simulink model "LMOpenLoop2"  (R2014a)
settings: Solver=ode45  StartTime=0.0  StopTime=5  MaxStep=0.0034  RelTol=1e-9
libraries: powerlib_meascontrol x2
settings Model: Creator=Daniel  LastModifiedBy=Daniel
settings SolverCC: ConsecutiveZCsStepRelTol=10*64*eps
settings DataIOCC: MaxDataPoints=200000  Refine=20

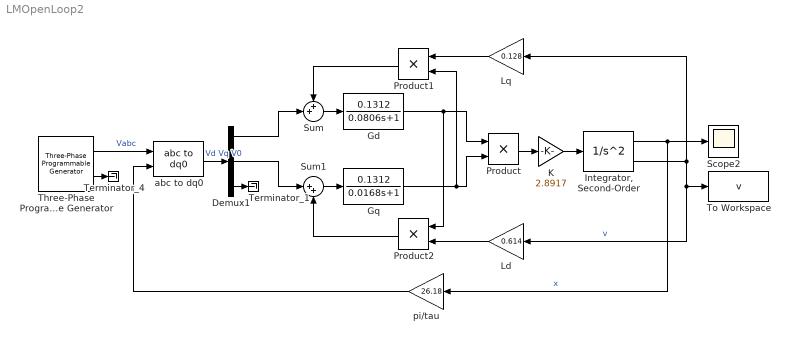
== system LMOpenLoop2 ==
  Demux1 : Demux  Outputs=3
  Gd : TransferFcn  Numerator=[0.1312]  Denominator=[0.0806 1]
  Gq : TransferFcn  Numerator=[0.1312]  Denominator=[0.0168 1]
  "Integrator, Second-Order" : SecondOrderIntegrator  ICDXDT=7.3495
  K : Gain  Gain=2.8917
  Ld : Gain  Gain=0.614
  Lq : Gain  Gain=0.128
  Product : Product
  Product1 : Product
  Product2 : Product
  Scope2 : Scope
      settings: ShowLegends=on
  Sum : Sum  Inputs=++|
  Sum1 : Sum  Inputs=|++
  Terminator_1 : Terminator
  Terminator_4 : Terminator
  Three-Phase Programmable Generator : powerlib_meascontrol/Pulse & Signal Generators/Three-Phase Programmable Generator  Par_Vps="[10.0  15  180/(2*pi)]"  VariationEntity=Amplitude  VariationType=Step  VariationStep=0  VariationRate=10  VariationMag=0.3  VariationFreq=2  Par_Timing_Variation=[0.5 1]  SinglePhase=on  Yampli=[1 0.2 1.2 1.0]  Xtime=[0 0.1 0.15 0.2]  HarmonicGeneration=off  Par_HarmoA=[1 0.3 -30 2]  Par_HarmoB=[1 0.0 0.0 1]  Par_Timing_Harmo="[0.1  1]"  Ts=50e-6
  To Workspace : ToWorkspace  VariableName=v  SaveFormat=Timeseries  SampleTime=-1
  abc to dq0 : powerlib_meascontrol/Transformations/abc to dq0  Alignment=Aligned with phase A axis
  pi/tau : Gain  Gain=26.18
  wires:
  Gd/1 -> Product/1, Product2/1
  Gq/1 -> Product1/2, Product/2
  Product/1 -> K/1
  "Integrator, Second-Order"/1 -> Scope2/1, pi/tau/1  "x"
  pi/tau/1 -> abc to dq0/2
  "Integrator, Second-Order"/2 -> To Workspace/1, Ld/1, Lq/1  "v"
  Demux1/1 -> Sum/2
  Lq/1 -> Product1/1
  Product1/1 -> Sum/1
  Sum/1 -> Gd/1
  Ld/1 -> Product2/2
  Demux1/2 -> Sum1/1
  Product2/1 -> Sum1/2
  Sum1/1 -> Gq/1
  K/1 -> "Integrator, Second-Order"/1
  Three-Phase Programmable Generator/2 -> Terminator_4/1
  Demux1/3 -> Terminator_1/1
  abc to dq0/1 -> Demux1/1  "Vd Vq V0"
  Three-Phase Programmable Generator/1 -> abc to dq0/1  "Vabc"
